simulink model "test_mdl_NI"  (R2018a)
settings: Solver=VariableStepAuto  StartTime=0.0  StopTime=10.0  RelTol=1e-3
(part 1 of 24)
settings Model: Creator=MSHI15  LastModifiedBy=MSHI15

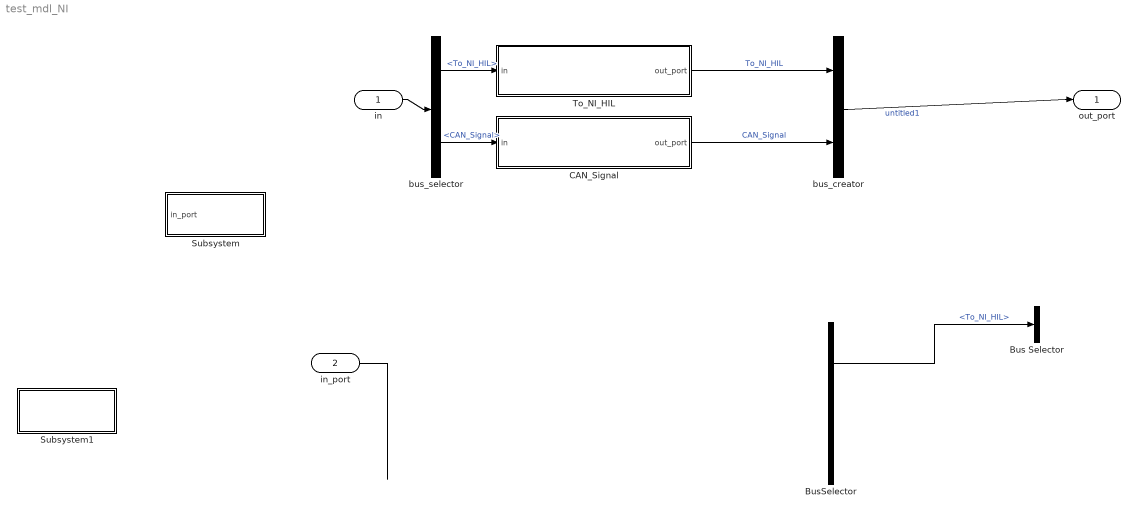
== system test_mdl_NI ==
  in : Inport
  in_port : Inport  Port=2
  Bus Selector : BusSelector  OutputSignals=signal1,signal2
  BusSelector : BusSelector  OutputSignals=To_NI_HIL,CAN_Signal
  CAN_Signal : Subsystem
  Subsystem : Subsystem
  Subsystem1 : Subsystem
  To_NI_HIL : Subsystem
  bus_creator : BusCreator  Inputs=2
  bus_selector : BusSelector  OutputSignals=To_NI_HIL,CAN_Signal
  out_port : Outport
  wires:
  BusSelector/1 -> Bus Selector/1  "<To_NI_HIL>"
  bus_creator/1 -> out_port/1  "untitled1"
  To_NI_HIL/1(out_port) -> bus_creator/1  "To_NI_HIL"
  CAN_Signal/1(out_port) -> bus_creator/2  "CAN_Signal"
  bus_selector/1 -> To_NI_HIL/1(in)  "<To_NI_HIL>"
  bus_selector/2 -> CAN_Signal/1(in)  "<CAN_Signal>"
  in/1 -> bus_selector/1
  in_port/1 -> ?

== system test_mdl_NI/CAN_Signal ==
  in : Inport
  ABS_ESC : Subsystem
  ADAS : Subsystem
  BCM : Subsystem
  DSMC : Subsystem
  ECM_DIESEL PCM PCM_HEV : Subsystem
  GWM : Subsystem
  PSCM : Subsystem
  RealPCM : Subsystem
  bus_creator : BusCreator  Inputs=8
  bus_selector : BusSelector  OutputSignals=ADAS,RealPCM,ABS_ESC,PSCM,ECM_DIESEL PCM PCM_HEV,BCM,GWM,DSMC
  out_port : Outport
  wires:
  bus_creator/1 -> out_port/1  "CAN_Signal"
  ADAS/1(out_port) -> bus_creator/1  "ADAS"
  RealPCM/1(out_port) -> bus_creator/2  "RealPCM"
  ABS_ESC/1(out_port) -> bus_creator/3  "ABS_ESC"
  PSCM/1(out_port) -> bus_creator/4  "PSCM"
  BCM/1(out_port) -> bus_creator/6  "BCM"
  GWM/1(out_port) -> bus_creator/7  "GWM"
  DSMC/1(out_port) -> bus_creator/8  "DSMC"
  ECM_DIESEL PCM PCM_HEV/1(out_port) -> bus_creator/5  "ECM_DIESEL PCM PCM_HEV"
  bus_selector/1 -> ADAS/1(in)  "<ADAS>"
  bus_selector/2 -> RealPCM/1(in)  "<RealPCM>"
  bus_selector/3 -> ABS_ESC/1(in)  "<ABS_ESC>"
  bus_selector/4 -> PSCM/1(in)  "<PSCM>"
  bus_selector/5 -> ECM_DIESEL PCM PCM_HEV/1(in)  "<ECM_DIESEL PCM PCM_HEV>"
  bus_selector/6 -> BCM/1(in)  "<BCM>"
  bus_selector/7 -> GWM/1(in)  "<GWM>"
  bus_selector/8 -> DSMC/1(in)  "<DSMC>"
  in/1 -> bus_selector/1

== system test_mdl_NI/Subsystem ==
  in_port : Inport
  ABS_ESC : Subsystem
  CMR_DSMC : Subsystem
  ECM_Diesel : Subsystem
  GWM : Subsystem
  IPMA_ADAS : Subsystem
  PCM : Subsystem
  PCM_HEV : Subsystem
  PSCM : Subsystem
  SOBDMC_HPCM_FD1 : Subsystem
  TCCM : Subsystem
  TCM_DSL : Subsystem
  TSTR : Subsystem
  VDM : Subsystem
  bus_selector : BusSelector  OutputSignals=ABS_ESC,CMR_DSMC,ECM_Diesel,GWM,IPMA_ADAS,PCM,PCM_HEV,PSCM,SOBDMC_HPCM_FD1,TCCM,TCM_DSL,TSTR,VDM
  wires:
  in_port/1 -> bus_selector/1  "Subsystem"
  bus_selector/1 -> ABS_ESC/1(in_port)  "<ABS_ESC>"
  bus_selector/2 -> CMR_DSMC/1(in_port)  "<CMR_DSMC>"
  bus_selector/3 -> ECM_Diesel/1(in_port)  "<ECM_Diesel>"
  bus_selector/4 -> GWM/1(in_port)  "<GWM>"
  bus_selector/5 -> IPMA_ADAS/1(in_port)  "<IPMA_ADAS>"
  bus_selector/6 -> PCM/1(in_port)  "<PCM>"
  bus_selector/7 -> PCM_HEV/1(in_port)  "<PCM_HEV>"
  bus_selector/8 -> PSCM/1(in_port)  "<PSCM>"
  bus_selector/9 -> SOBDMC_HPCM_FD1/1(in_port)  "<SOBDMC_HPCM_FD1>"
  bus_selector/10 -> TCCM/1(in_port)  "<TCCM>"
  bus_selector/11 -> TCM_DSL/1(in_port)  "<TCM_DSL>"
  bus_selector/12 -> TSTR/1(in_port)  "<TSTR>"
  bus_selector/13 -> VDM/1(in_port)  "<VDM>"

== system test_mdl_NI/Subsystem1 ==

== system test_mdl_NI/To_NI_HIL ==
  in : Inport
  DSMC : Subsystem
  MRR : Subsystem
  SRR_L : Subsystem
  SRR_R : Subsystem
  Soft_ABS : Subsystem
  Soft_APIM : Subsystem
  Soft_BCM : Subsystem
  Soft_CCM : Subsystem
  Soft_ECM : Subsystem
  Soft_IPC : Subsystem
  Soft_IPMA : Subsystem
  Soft_MRR : Subsystem
  Soft_PCM : Subsystem
  Soft_PSCM : Subsystem
  Soft_RCM : Subsystem
  Soft_SCCM : Subsystem
  Soft_TCM : Subsystem
  bus_creator : BusCreator  Inputs=17
  bus_selector : BusSelector  OutputSignals=Soft_ABS,Soft_PCM,Soft_ECM,Soft_TCM,Soft_PSCM,Soft_RCM,Soft_SCCM,Soft_MRR,Soft_BCM,Soft_IPC,Soft_APIM,Soft_IPMA,Soft_CCM,MRR,SRR_R,SRR_L,DSMC
  out_port : Outport
  wires:
  bus_creator/1 -> out_port/1  "To_NI_HIL"
  Soft_IPC/1(out) -> bus_creator/10  "Soft_IPC"
  Soft_APIM/1(out) -> bus_creator/11  "Soft_APIM"
  Soft_IPMA/1(out) -> bus_creator/12  "Soft_IPMA"
  Soft_CCM/1(out) -> bus_creator/13  "Soft_CCM"
  Soft_ABS/1(out_port) -> bus_creator/1  "Soft_ABS"
  Soft_PCM/1(out_port) -> bus_creator/2  "Soft_PCM"
  Soft_ECM/1(out_port) -> bus_creator/3  "Soft_ECM"
  Soft_TCM/1(out_port) -> bus_creator/4  "Soft_TCM"
  Soft_PSCM/1(out_port) -> bus_creator/5  "Soft_PSCM"
  Soft_RCM/1(out_port) -> bus_creator/6  "Soft_RCM"
  Soft_SCCM/1(out_port) -> bus_creator/7  "Soft_SCCM"
  Soft_MRR/1(out_port) -> bus_creator/8  "Soft_MRR"
  Soft_BCM/1(out_port) -> bus_creator/9  "Soft_BCM"
  MRR/1(out_port) -> bus_creator/14  "MRR"
  SRR_R/1(out_port) -> bus_creator/15  "SRR_R"
  SRR_L/1(out_port) -> bus_creator/16  "SRR_L"
  DSMC/1(out_port) -> bus_creator/17  "DSMC"
  bus_selector/1 -> Soft_ABS/1(in)  "<Soft_ABS>"
  bus_selector/2 -> Soft_PCM/1(in)  "<Soft_PCM>"
  bus_selector/3 -> Soft_ECM/1(in)  "<Soft_ECM>"
  bus_selector/4 -> Soft_TCM/1(in)  "<Soft_TCM>"
  bus_selector/5 -> Soft_PSCM/1(in)  "<Soft_PSCM>"
  bus_selector/6 -> Soft_RCM/1(in)  "<Soft_RCM>"
  bus_selector/7 -> Soft_SCCM/1(in)  "<Soft_SCCM>"
  bus_selector/8 -> Soft_MRR/1(in)  "<Soft_MRR>"
  bus_selector/9 -> Soft_BCM/1(in)  "<Soft_BCM>"
  bus_selector/10 -> Soft_IPC/1(in)  "<Soft_IPC>"
  bus_selector/11 -> Soft_APIM/1(in)  "<Soft_APIM>"
  bus_selector/12 -> Soft_IPMA/1(in)  "<Soft_IPMA>"
  bus_selector/13 -> Soft_CCM/1(in)  "<Soft_CCM>"
  bus_selector/14 -> MRR/1(in)  "<MRR>"
  bus_selector/15 -> SRR_R/1(in)  "<SRR_R>"
  bus_selector/16 -> SRR_L/1(in)  "<SRR_L>"
  bus_selector/17 -> DSMC/1(in)  "<DSMC>"
  in/1 -> bus_selector/1

== system test_mdl_NI/CAN_Signal/ABS_ESC ==
  in : Inport
  ABS_AutoSar_NetworkMgt_0x596 : Subsystem
  ABS_BrkBst_Data_0x4B0 : Subsystem
  ABS_Rapid_Data_Response_1_0x6B0 : Subsystem
  ABS_Rapid_Data_Response_2_0x6B1 : Subsystem
  ActiveFronSteering_Req_0x88 : Subsystem
  BrakeSnData_3_0x77 : Subsystem
  BrakeSnData_4_0x7D : Subsystem
  BrakeSnData_5_0x76 : Subsystem
  BrakeSnData_6_0x414 : Subsystem
  BrakeSysFeatures_0x415 : Subsystem
  BrakeSysFeatures_2_0x416 : Subsystem
  BrakeSysFeatures_3_0x41E : Subsystem
  DesiredTorqBrk_0x213 : Subsystem
  DesiredTorqBrk_2_0x214 : Subsystem
  Global_PATS_SubTarget_0x49 : Subsystem
  SelectDriveModeData2_0x44E : Subsystem
  SelectDriveModeData_0x420 : Subsystem
  SteeringPinion_Data2_0x7F : Subsystem
  TesterPhysicalResABS_0x768 : Subsystem
  TrailerBrakeData_0x412 : Subsystem
  WheelData_0x216 : Subsystem
  WheelSpeed_0x217 : Subsystem
  bus_creator : BusCreator  Inputs=22
  bus_selector : BusSelector  OutputSignals=Global_PATS_SubTarget_0x49,BrakeSnData_5_0x76,BrakeSnData_3_0x77,BrakeSnData_4_0x7D,SteeringPinion_Data2_0x7F,ActiveFronSteering_Req_0x88,DesiredTorqBrk_0x213,DesiredTorqBrk_2_0x214,WheelData_0x216,WheelSpeed_0x217,TrailerBrakeData_0x412,BrakeSnData_6_0x414,BrakeSysFeatures_0x415,BrakeSysFeatures_2_0x416,BrakeSysFeatures_3_0x41E,SelectDriveModeData_0x420,SelectDriveModeData2_0x44E,ABS_BrkBst_Data_0x4B0,ABS_AutoSar_NetworkMgt_0x596,ABS_Rapid_Data_Response_1_0x6B0,ABS_Rapid_Data_Response_2_0x6B1,TesterPhysicalResABS_0x768
  out_port : Outport
  wires:
  bus_creator/1 -> out_port/1  "ABS_ESC"
  Global_PATS_SubTarget_0x49/1(out_port) -> bus_creator/1  "Global_PATS_SubTarget_0x49"
  BrakeSnData_5_0x76/1(out_port) -> bus_creator/2  "BrakeSnData_5_0x76"
  BrakeSnData_3_0x77/1(out_port) -> bus_creator/3  "BrakeSnData_3_0x77"
  BrakeSnData_4_0x7D/1(out_port) -> bus_creator/4  "BrakeSnData_4_0x7D"
  SteeringPinion_Data2_0x7F/1(out_port) -> bus_creator/5  "SteeringPinion_Data2_0x7F"
  ActiveFronSteering_Req_0x88/1(out_port) -> bus_creator/6  "ActiveFronSteering_Req_0x88"
  DesiredTorqBrk_0x213/1(out_port) -> bus_creator/7  "DesiredTorqBrk_0x213"
  DesiredTorqBrk_2_0x214/1(out_port) -> bus_creator/8  "DesiredTorqBrk_2_0x214"
  WheelData_0x216/1(out_port) -> bus_creator/9  "WheelData_0x216"
  WheelSpeed_0x217/1(out_port) -> bus_creator/10  "WheelSpeed_0x217"
  TrailerBrakeData_0x412/1(out_port) -> bus_creator/11  "TrailerBrakeData_0x412"
  BrakeSnData_6_0x414/1(out_port) -> bus_creator/12  "BrakeSnData_6_0x414"
  BrakeSysFeatures_0x415/1(out_port) -> bus_creator/13  "BrakeSysFeatures_0x415"
  BrakeSysFeatures_2_0x416/1(out_port) -> bus_creator/14  "BrakeSysFeatures_2_0x416"
  BrakeSysFeatures_3_0x41E/1(out_port) -> bus_creator/15  "BrakeSysFeatures_3_0x41E"
  SelectDriveModeData_0x420/1(out_port) -> bus_creator/16  "SelectDriveModeData_0x420"
  SelectDriveModeData2_0x44E/1(out_port) -> bus_creator/17  "SelectDriveModeData2_0x44E"
  ABS_BrkBst_Data_0x4B0/1(out_port) -> bus_creator/18  "ABS_BrkBst_Data_0x4B0"
  ABS_AutoSar_NetworkMgt_0x596/1(out_port) -> bus_creator/19  "ABS_AutoSar_NetworkMgt_0x596"
  ABS_Rapid_Data_Response_1_0x6B0/1(out_port) -> bus_creator/20  "ABS_Rapid_Data_Response_1_0x6B0"
  ABS_Rapid_Data_Response_2_0x6B1/1(out_port) -> bus_creator/21  "ABS_Rapid_Data_Response_2_0x6B1"
  TesterPhysicalResABS_0x768/1(out_port) -> bus_creator/22  "TesterPhysicalResABS_0x768"
  bus_selector/1 -> Global_PATS_SubTarget_0x49/1(in)  "<Global_PATS_SubTarget_0x49>"
  bus_selector/2 -> BrakeSnData_5_0x76/1(in)  "<BrakeSnData_5_0x76>"
  bus_selector/3 -> BrakeSnData_3_0x77/1(in)  "<BrakeSnData_3_0x77>"
  bus_selector/4 -> BrakeSnData_4_0x7D/1(in)  "<BrakeSnData_4_0x7D>"
  bus_selector/5 -> SteeringPinion_Data2_0x7F/1(in)  "<SteeringPinion_Data2_0x7F>"
  bus_selector/6 -> ActiveFronSteering_Req_0x88/1(in)  "<ActiveFronSteering_Req_0x88>"
  bus_selector/7 -> DesiredTorqBrk_0x213/1(in)  "<DesiredTorqBrk_0x213>"
  bus_selector/8 -> DesiredTorqBrk_2_0x214/1(in)  "<DesiredTorqBrk_2_0x214>"
  bus_selector/9 -> WheelData_0x216/1(in)  "<WheelData_0x216>"
  bus_selector/10 -> WheelSpeed_0x217/1(in)  "<WheelSpeed_0x217>"
  bus_selector/11 -> TrailerBrakeData_0x412/1(in)  "<TrailerBrakeData_0x412>"
  bus_selector/12 -> BrakeSnData_6_0x414/1(in)  "<BrakeSnData_6_0x414>"
  bus_selector/13 -> BrakeSysFeatures_0x415/1(in)  "<BrakeSysFeatures_0x415>"
  bus_selector/14 -> BrakeSysFeatures_2_0x416/1(in)  "<BrakeSysFeatures_2_0x416>"
  bus_selector/15 -> BrakeSysFeatures_3_0x41E/1(in)  "<BrakeSysFeatures_3_0x41E>"
  bus_selector/16 -> SelectDriveModeData_0x420/1(in)  "<SelectDriveModeData_0x420>"
  bus_selector/17 -> SelectDriveModeData2_0x44E/1(in)  "<SelectDriveModeData2_0x44E>"
  bus_selector/18 -> ABS_BrkBst_Data_0x4B0/1(in)  "<ABS_BrkBst_Data_0x4B0>"
  bus_selector/19 -> ABS_AutoSar_NetworkMgt_0x596/1(in)  "<ABS_AutoSar_NetworkMgt_0x596>"
  bus_selector/20 -> ABS_Rapid_Data_Response_1_0x6B0/1(in)  "<ABS_Rapid_Data_Response_1_0x6B0>"
  bus_selector/21 -> ABS_Rapid_Data_Response_2_0x6B1/1(in)  "<ABS_Rapid_Data_Response_2_0x6B1>"
  bus_selector/22 -> TesterPhysicalResABS_0x768/1(in)  "<TesterPhysicalResABS_0x768>"
  in/1 -> bus_selector/1

== system test_mdl_NI/CAN_Signal/ADAS ==
  in : Inport
  ACCDATA : Subsystem
  ACCDATA_2 : Subsystem
  bus_creator : BusCreator  Inputs=2
  bus_selector : BusSelector  OutputSignals=ACCDATA,ACCDATA_2
  out_port : Outport
  wires:
  bus_creator/1 -> out_port/1  "ADAS"
  ACCDATA/1(out_port) -> bus_creator/1  "ACCDATA"
  ACCDATA_2/1(out_port) -> bus_creator/2  "ACCDATA_2"
  bus_selector/1 -> ACCDATA/1(in)  "<ACCDATA>"
  bus_selector/2 -> ACCDATA_2/1(in)  "<ACCDATA_2>"
  in/1 -> bus_selector/1

== system test_mdl_NI/CAN_Signal/BCM ==
  in : Inport
  BCM_Lamp_Stat_0x3C3 : Subsystem
  Battery_Mgmt_24V_0x42E : Subsystem
  Battery_Mgmt_2_0x42C : Subsystem
  Battery_Mgmt_3_0x43C : Subsystem
  Battery_Mgmt_4_0x42B : Subsystem
  BodyInfo_3_0x3B3 : Subsystem
  Body_Info_10_0x3BA : Subsystem
  Body_Info_12_0x26E : Subsystem
  Body_Info_4_0x242 : Subsystem
  Body_Info_6_0x38D : Subsystem
  Body_Info_7_0x3B1 : Subsystem
  Body_Info_8_0x3B9 : Subsystem
  Body_Info_9_0x3A3 : Subsystem
  CMPS_FDM_Info_Status_0x3C7 : Subsystem
  CellPhonePassport_Stat_1_0x447 : Subsystem
  GGCC_Config_Mgmt_ID_1_0x40A : Subsystem
  GlobalClock_Data_0x84 : Subsystem
  Global_PATS_Control_Info2_0x42 : Subsystem
  Global_PATS_Control_Info_0x41 : Subsystem
  Locking_Systems_2_0x331 : Subsystem
  PaakRqData1_0x468 : Subsystem
  PaakRqData2_0x469 : Subsystem
  Personality_BCM2_Data_0x3EB : Subsystem
  Personality_BCM_Data_0x3E3 : Subsystem
  Power_Stat_0x456 : Subsystem
  RKE_Packet_0x3B6 : Subsystem
  TPM_Frame_0x3B7 : Subsystem
  Tire_Pressure_Data_0x3B5 : Subsystem
  Tire_Pressure_Data_DRW_0x3B8 : Subsystem
  Tire_Pressure_Stat_0x3B4 : Subsystem
  bus_creator : BusCreator  Inputs=30
  bus_selector : BusSelector  OutputSignals=Global_PATS_Control_Info_0x41,Global_PATS_Control_Info2_0x42,GlobalClock_Data_0x84,Body_Info_4_0x242,Body_Info_12_0x26E,Locking_Systems_2_0x331,Body_Info_6_0x38D,Body_Info_9_0x3A3,Body_Info_7_0x3B1,BodyInfo_3_0x3B3,Tire_Pressure_Stat_0x3B4,Tire_Pressure_Data_0x3B5,RKE_Packet_0x3B6,TPM_Frame_0x3B7,Tire_Pressure_Data_DRW_0x3B8,Body_Info_8_0x3B9,Body_Info_10_0x3BA,BCM_Lamp_Stat_0x3C3,CMPS_FDM_Info_Status_0x3C7,Personality_BCM_Data_0x3E3,Personality_BCM2_Data_0x3EB,GGCC_Config_Mgmt_ID_1_0x40A,Battery_Mgmt_4_0x42B,Battery_Mgmt_2_0x42C,Battery_Mgmt_24V_0x42E,Battery_Mgmt_3_0x43C,CellPhonePassport_Stat_1_0x447,Power_Stat_0x456,PaakRqData1_0x468,PaakRqData2_0x469
  out_port : Outport
  wires:
  bus_creator/1 -> out_port/1  "BCM"
  Global_PATS_Control_Info_0x41/1(out_port) -> bus_creator/1  "Global_PATS_Control_Info_0x41"
  Global_PATS_Control_Info2_0x42/1(out_port) -> bus_creator/2  "Global_PATS_Control_Info2_0x42"
  GlobalClock_Data_0x84/1(out_port) -> bus_creator/3  "GlobalClock_Data_0x84"
  Body_Info_4_0x242/1(out_port) -> bus_creator/4  "Body_Info_4_0x242"
  Body_Info_12_0x26E/1(out_port) -> bus_creator/5  "Body_Info_12_0x26E"
  Locking_Systems_2_0x331/1(out_port) -> bus_creator/6  "Locking_Systems_2_0x331"
  Body_Info_6_0x38D/1(out_port) -> bus_creator/7  "Body_Info_6_0x38D"
  Body_Info_9_0x3A3/1(out_port) -> bus_creator/8  "Body_Info_9_0x3A3"
  Body_Info_7_0x3B1/1(out_port) -> bus_creator/9  "Body_Info_7_0x3B1"
  BodyInfo_3_0x3B3/1(out_port) -> bus_creator/10  "BodyInfo_3_0x3B3"
  Tire_Pressure_Stat_0x3B4/1(out_port) -> bus_creator/11  "Tire_Pressure_Stat_0x3B4"
  Tire_Pressure_Data_0x3B5/1(out_port) -> bus_creator/12  "Tire_Pressure_Data_0x3B5"
  RKE_Packet_0x3B6/1(out_port) -> bus_creator/13  "RKE_Packet_0x3B6"
  TPM_Frame_0x3B7/1(out_port) -> bus_creator/14  "TPM_Frame_0x3B7"
  Tire_Pressure_Data_DRW_0x3B8/1(out_port) -> bus_creator/15  "Tire_Pressure_Data_DRW_0x3B8"
  Body_Info_8_0x3B9/1(out_port) -> bus_creator/16  "Body_Info_8_0x3B9"
  Body_Info_10_0x3BA/1(out_port) -> bus_creator/17  "Body_Info_10_0x3BA"
  BCM_Lamp_Stat_0x3C3/1(out_port) -> bus_creator/18  "BCM_Lamp_Stat_0x3C3"
  CMPS_FDM_Info_Status_0x3C7/1(out_port) -> bus_creator/19  "CMPS_FDM_Info_Status_0x3C7"
  Personality_BCM_Data_0x3E3/1(out_port) -> bus_creator/20  "Personality_BCM_Data_0x3E3"
  Personality_BCM2_Data_0x3EB/1(out_port) -> bus_creator/21  "Personality_BCM2_Data_0x3EB"
  GGCC_Config_Mgmt_ID_1_0x40A/1(out_port) -> bus_creator/22  "GGCC_Config_Mgmt_ID_1_0x40A"
  Battery_Mgmt_4_0x42B/1(out_port) -> bus_creator/23  "Battery_Mgmt_4_0x42B"
  Battery_Mgmt_2_0x42C/1(out_port) -> bus_creator/24  "Battery_Mgmt_2_0x42C"
  Battery_Mgmt_24V_0x42E/1(out_port) -> bus_creator/25  "Battery_Mgmt_24V_0x42E"
  Battery_Mgmt_3_0x43C/1(out_port) -> bus_creator/26  "Battery_Mgmt_3_0x43C"
  CellPhonePassport_Stat_1_0x447/1(out_port) -> bus_creator/27  "CellPhonePassport_Stat_1_0x447"
  Power_Stat_0x456/1(out_port) -> bus_creator/28  "Power_Stat_0x456"
  PaakRqData1_0x468/1(out_port) -> bus_creator/29  "PaakRqData1_0x468"
  PaakRqData2_0x469/1(out_port) -> bus_creator/30  "PaakRqData2_0x469"
  bus_selector/1 -> Global_PATS_Control_Info_0x41/1(in)  "<Global_PATS_Control_Info_0x41>"
  bus_selector/2 -> Global_PATS_Control_Info2_0x42/1(in)  "<Global_PATS_Control_Info2_0x42>"
  bus_selector/3 -> GlobalClock_Data_0x84/1(in)  "<GlobalClock_Data_0x84>"
  bus_selector/4 -> Body_Info_4_0x242/1(in)  "<Body_Info_4_0x242>"
  bus_selector/5 -> Body_Info_12_0x26E/1(in)  "<Body_Info_12_0x26E>"
  bus_selector/6 -> Locking_Systems_2_0x331/1(in)  "<Locking_Systems_2_0x331>"
  bus_selector/7 -> Body_Info_6_0x38D/1(in)  "<Body_Info_6_0x38D>"
  bus_selector/8 -> Body_Info_9_0x3A3/1(in)  "<Body_Info_9_0x3A3>"
  bus_selector/9 -> Body_Info_7_0x3B1/1(in)  "<Body_Info_7_0x3B1>"
  bus_selector/10 -> BodyInfo_3_0x3B3/1(in)  "<BodyInfo_3_0x3B3>"
  bus_selector/11 -> Tire_Pressure_Stat_0x3B4/1(in)  "<Tire_Pressure_Stat_0x3B4>"
  bus_selector/12 -> Tire_Pressure_Data_0x3B5/1(in)  "<Tire_Pressure_Data_0x3B5>"
  bus_selector/13 -> RKE_Packet_0x3B6/1(in)  "<RKE_Packet_0x3B6>"
  bus_selector/14 -> TPM_Frame_0x3B7/1(in)  "<TPM_Frame_0x3B7>"
  bus_selector/15 -> Tire_Pressure_Data_DRW_0x3B8/1(in)  "<Tire_Pressure_Data_DRW_0x3B8>"
  bus_selector/16 -> Body_Info_8_0x3B9/1(in)  "<Body_Info_8_0x3B9>"
  bus_selector/17 -> Body_Info_10_0x3BA/1(in)  "<Body_Info_10_0x3BA>"
  bus_selector/18 -> BCM_Lamp_Stat_0x3C3/1(in)  "<BCM_Lamp_Stat_0x3C3>"
  bus_selector/19 -> CMPS_FDM_Info_Status_0x3C7/1(in)  "<CMPS_FDM_Info_Status_0x3C7>"
  bus_selector/20 -> Personality_BCM_Data_0x3E3/1(in)  "<Personality_BCM_Data_0x3E3>"
  bus_selector/21 -> Personality_BCM2_Data_0x3EB/1(in)  "<Personality_BCM2_Data_0x3EB>"
  bus_selector/22 -> GGCC_Config_Mgmt_ID_1_0x40A/1(in)  "<GGCC_Config_Mgmt_ID_1_0x40A>"
  bus_selector/23 -> Battery_Mgmt_4_0x42B/1(in)  "<Battery_Mgmt_4_0x42B>"
  bus_selector/24 -> Battery_Mgmt_2_0x42C/1(in)  "<Battery_Mgmt_2_0x42C>"
  bus_selector/25 -> Battery_Mgmt_24V_0x42E/1(in)  "<Battery_Mgmt_24V_0x42E>"
  bus_selector/26 -> Battery_Mgmt_3_0x43C/1(in)  "<Battery_Mgmt_3_0x43C>"
  bus_selector/27 -> CellPhonePassport_Stat_1_0x447/1(in)  "<CellPhonePassport_Stat_1_0x447>"
  bus_selector/28 -> Power_Stat_0x456/1(in)  "<Power_Stat_0x456>"
  bus_selector/29 -> PaakRqData1_0x468/1(in)  "<PaakRqData1_0x468>"
  bus_selector/30 -> PaakRqData2_0x469/1(in)  "<PaakRqData2_0x469>"
  in/1 -> bus_selector/1

== system test_mdl_NI/CAN_Signal/DSMC ==
  in : Inport
  CMR_DSMC_AutoSar_NetwrkMgt : Subsystem
  DrvStatMonData : Subsystem
  TesterPhysicalResCMR_DSMC : Subsystem
  bus_creator : BusCreator  Inputs=3
  bus_selector : BusSelector  OutputSignals=CMR_DSMC_AutoSar_NetwrkMgt,DrvStatMonData,TesterPhysicalResCMR_DSMC
  out_port : Outport
  wires:
  bus_creator/1 -> out_port/1  "DSMC"
  CMR_DSMC_AutoSar_NetwrkMgt/1(out_port) -> bus_creator/1  "CMR_DSMC_AutoSar_NetwrkMgt"
  DrvStatMonData/1(out_port) -> bus_creator/2  "DrvStatMonData"
  TesterPhysicalResCMR_DSMC/1(out_port) -> bus_creator/3  "TesterPhysicalResCMR_DSMC"
  bus_selector/1 -> CMR_DSMC_AutoSar_NetwrkMgt/1(in)  "<CMR_DSMC_AutoSar_NetwrkMgt>"
  bus_selector/2 -> DrvStatMonData/1(in)  "<DrvStatMonData>"
  bus_selector/3 -> TesterPhysicalResCMR_DSMC/1(in)  "<TesterPhysicalResCMR_DSMC>"
  in/1 -> bus_selector/1

== system test_mdl_NI/CAN_Signal/ECM_DIESEL PCM PCM_HEV ==
  in : Inport
  EngBrakeData_0x165 : Subsystem
  EngVehicleSpThrottle2_0x202 : Subsystem
  EngVehicleSpThrottle_0x204 : Subsystem
  EngineClimateData_0x178 : Subsystem
  EngineData_6_0x156 : Subsystem
  EngineData_7_0x179 : Subsystem
  Engine_Clutch_Data_0x42F : Subsystem
  Gear_Shift_by_Wire_3 : Subsystem
  Global_PATS_TargetInfo_0x47 : Subsystem
  HEV_Powertrain_Data2 : Subsystem
  PCM_AutoSar_NetworkMgmt_0x595 : Subsystem
  PCM_Rapid_Data_Response_1_0x6A0 : Subsystem
  PowertrainData_10 : Subsystem
  PowertrainData_1_0x421 : Subsystem
  PowertrainData_2_0x42D : Subsystem
  PowertrainData_3_0x43E : Subsystem
  PowertrainData_6_0x205 : Subsystem
  PowertrainData_7_0x41F : Subsystem
  PowertrainData_9_0x44C : Subsystem
  Powertrain_Data_4_0x424 : Subsystem
  Powertrain_Data_5_0x43F : Subsystem
  Stop_Start_0x166 : Subsystem
  TesterPhysicalResPCM_0x7E8 : Subsystem
  TorqueDataEngFlags_0x200 : Subsystem
  TransGearData : Subsystem
  VehicleOperatingModes_0x167 : Subsystem
  bus_creator : BusCreator  Inputs=26
  bus_selector : BusSelector  OutputSignals=Global_PATS_TargetInfo_0x47,EngineData_6_0x156,EngBrakeData_0x165,Stop_Start_0x166,VehicleOperatingModes_0x167,EngineClimateData_0x178,EngineData_7_0x179,TorqueDataEngFlags_0x200,EngVehicleSpThrottle2_0x202,EngVehicleSpThrottle_0x204,PowertrainData_6_0x205,PowertrainData_7_0x41F,PowertrainData_1_0x421,Powertrain_Data_4_0x424,PowertrainData_2_0x42D,Engine_Clutch_Data_0x42F,PowertrainData_3_0x43E,Powertrain_Data_5_0x43F,PowertrainData_9_0x44C,PCM_AutoSar_NetworkMgmt_0x595,PCM_Rapid_Data_Response_1_0x6A0,TesterPhysicalResPCM_0x7E8,Gear_Shift_by_Wire_3,PowertrainData_10,TransGearData,HEV_Powertrain_Data2
  out_port : Outport
  wires:
  bus_creator/1 -> out_port/1  "ECM_DIESEL PCM PCM_HEV"
  Global_PATS_TargetInfo_0x47/1(out_port) -> bus_creator/1  "Global_PATS_TargetInfo_0x47"
  EngineData_6_0x156/1(out_port) -> bus_creator/2  "EngineData_6_0x156"
  EngBrakeData_0x165/1(out_port) -> bus_creator/3  "EngBrakeData_0x165"
  Stop_Start_0x166/1(out_port) -> bus_creator/4  "Stop_Start_0x166"
  VehicleOperatingModes_0x167/1(out_port) -> bus_creator/5  "VehicleOperatingModes_0x167"
  EngineClimateData_0x178/1(out_port) -> bus_creator/6  "EngineClimateData_0x178"
  EngineData_7_0x179/1(out_port) -> bus_creator/7  "EngineData_7_0x179"
  TorqueDataEngFlags_0x200/1(out_port) -> bus_creator/8  "TorqueDataEngFlags_0x200"
  EngVehicleSpThrottle2_0x202/1(out_port) -> bus_creator/9  "EngVehicleSpThrottle2_0x202"
  EngVehicleSpThrottle_0x204/1(out_port) -> bus_creator/10  "EngVehicleSpThrottle_0x204"
  PowertrainData_6_0x205/1(out_port) -> bus_creator/11  "PowertrainData_6_0x205"
  PowertrainData_7_0x41F/1(out_port) -> bus_creator/12  "PowertrainData_7_0x41F"
  PowertrainData_1_0x421/1(out_port) -> bus_creator/13  "PowertrainData_1_0x421"
  Powertrain_Data_4_0x424/1(out_port) -> bus_creator/14  "Powertrain_Data_4_0x424"
  PowertrainData_2_0x42D/1(out_port) -> bus_creator/15  "PowertrainData_2_0x42D"
  Engine_Clutch_Data_0x42F/1(out_port) -> bus_creator/16  "Engine_Clutch_Data_0x42F"
  PowertrainData_3_0x43E/1(out_port) -> bus_creator/17  "PowertrainData_3_0x43E"
  Powertrain_Data_5_0x43F/1(out_port) -> bus_creator/18  "Powertrain_Data_5_0x43F"
  PowertrainData_9_0x44C/1(out_port) -> bus_creator/19  "PowertrainData_9_0x44C"
  PCM_AutoSar_NetworkMgmt_0x595/1(out_port) -> bus_creator/20  "PCM_AutoSar_NetworkMgmt_0x595"
  PCM_Rapid_Data_Response_1_0x6A0/1(out_port) -> bus_creator/21  "PCM_Rapid_Data_Response_1_0x6A0"
  TesterPhysicalResPCM_0x7E8/1(out_port) -> bus_creator/22  "TesterPhysicalResPCM_0x7E8"
  Gear_Shift_by_Wire_3/1(out_port) -> bus_creator/23  "Gear_Shift_by_Wire_3"
  PowertrainData_10/1(out_port) -> bus_creator/24  "PowertrainData_10"
  TransGearData/1(out_port) -> bus_creator/25  "TransGearData"
  HEV_Powertrain_Data2/1(out_port) -> bus_creator/26  "HEV_Powertrain_Data2"
  bus_selector/1 -> Global_PATS_TargetInfo_0x47/1(in)  "<Global_PATS_TargetInfo_0x47>"
  bus_selector/2 -> EngineData_6_0x156/1(in)  "<EngineData_6_0x156>"
  bus_selector/3 -> EngBrakeData_0x165/1(in)  "<EngBrakeData_0x165>"
  bus_selector/4 -> Stop_Start_0x166/1(in)  "<Stop_Start_0x166>"
  bus_selector/5 -> VehicleOperatingModes_0x167/1(in)  "<VehicleOperatingModes_0x167>"
  bus_selector/6 -> EngineClimateData_0x178/1(in)  "<EngineClimateData_0x178>"
  bus_selector/7 -> EngineData_7_0x179/1(in)  "<EngineData_7_0x179>"
  bus_selector/8 -> TorqueDataEngFlags_0x200/1(in)  "<TorqueDataEngFlags_0x200>"
  bus_selector/9 -> EngVehicleSpThrottle2_0x202/1(in)  "<EngVehicleSpThrottle2_0x202>"
  bus_selector/10 -> EngVehicleSpThrottle_0x204/1(in)  "<EngVehicleSpThrottle_0x204>"
  bus_selector/11 -> PowertrainData_6_0x205/1(in)  "<PowertrainData_6_0x205>"
  bus_selector/12 -> PowertrainData_7_0x41F/1(in)  "<PowertrainData_7_0x41F>"
  bus_selector/13 -> PowertrainData_1_0x421/1(in)  "<PowertrainData_1_0x421>"
  bus_selector/14 -> Powertrain_Data_4_0x424/1(in)  "<Powertrain_Data_4_0x424>"
  bus_selector/15 -> PowertrainData_2_0x42D/1(in)  "<PowertrainData_2_0x42D>"
  bus_selector/16 -> Engine_Clutch_Data_0x42F/1(in)  "<Engine_Clutch_Data_0x42F>"
  bus_selector/17 -> PowertrainData_3_0x43E/1(in)  "<PowertrainData_3_0x43E>"
  bus_selector/18 -> Powertrain_Data_5_0x43F/1(in)  "<Powertrain_Data_5_0x43F>"
  bus_selector/19 -> PowertrainData_9_0x44C/1(in)  "<PowertrainData_9_0x44C>"
  bus_selector/20 -> PCM_AutoSar_NetworkMgmt_0x595/1(in)  "<PCM_AutoSar_NetworkMgmt_0x595>"
  bus_selector/21 -> PCM_Rapid_Data_Response_1_0x6A0/1(in)  "<PCM_Rapid_Data_Response_1_0x6A0>"
  bus_selector/22 -> TesterPhysicalResPCM_0x7E8/1(in)  "<TesterPhysicalResPCM_0x7E8>"
  bus_selector/23 -> Gear_Shift_by_Wire_3/1(in)  "<Gear_Shift_by_Wire_3>"
  bus_selector/24 -> PowertrainData_10/1(in)  "<PowertrainData_10>"
  bus_selector/25 -> TransGearData/1(in)  "<TransGearData>"
  bus_selector/26 -> HEV_Powertrain_Data2/1(in)  "<HEV_Powertrain_Data2>"
  in/1 -> bus_selector/1

== system test_mdl_NI/CAN_Signal/GWM ==
  in : Inport
  GSM : Subsystem
  Other_GWMTx : Subsystem
  RCM : Subsystem
  SCCM : Subsystem
  Tester_AutoSar : Subsystem
  bus_creator : BusCreator  Inputs=5
  bus_selector : BusSelector  OutputSignals=Other_GWMTx,RCM,SCCM,GSM,Tester_AutoSar
  out_port : Outport
  wires:
  bus_creator/1 -> out_port/1  "GWM"
  Other_GWMTx/1(out_port) -> bus_creator/1  "Other_GWMTx"
  RCM/1(out_port) -> bus_creator/2  "RCM"
  SCCM/1(out_port) -> bus_creator/3  "SCCM"
  GSM/1(out_port) -> bus_creator/4  "GSM"
  Tester_AutoSar/1(out_port) -> bus_creator/5  "Tester_AutoSar"
  bus_selector/1 -> Other_GWMTx/1(in)  "<Other_GWMTx>"
  bus_selector/2 -> RCM/1(in)  "<RCM>"
  bus_selector/3 -> SCCM/1(in)  "<SCCM>"
  bus_selector/4 -> GSM/1(in)  "<GSM>"
  bus_selector/5 -> Tester_AutoSar/1(in)  "<Tester_AutoSar>"
  in/1 -> bus_selector/1

== system test_mdl_NI/CAN_Signal/PSCM ==
  in : Inport
  EPAS_INFO_0x82 : Subsystem
  Lane_Assist_Data3_FD1_0x3CC : Subsystem
  PSCM_AutoSar_NetwrkMgmt_0x5B5 : Subsystem
  SteeringPinion_Data_0x7E : Subsystem
  TesterPhysicalResPSCM_0x738 : Subsystem
  TrailerAid_Data2_0x417 : Subsystem
  bus_creator : BusCreator  Inputs=6
  bus_selector : BusSelector  OutputSignals=SteeringPinion_Data_0x7E,EPAS_INFO_0x82,Lane_Assist_Data3_FD1_0x3CC,TrailerAid_Data2_0x417,PSCM_AutoSar_NetwrkMgmt_0x5B5,TesterPhysicalResPSCM_0x738
  out_port : Outport
  wires:
  bus_creator/1 -> out_port/1  "PSCM"
  SteeringPinion_Data_0x7E/1(out_port) -> bus_creator/1  "SteeringPinion_Data_0x7E"
  EPAS_INFO_0x82/1(out_port) -> bus_creator/2  "EPAS_INFO_0x82"
  Lane_Assist_Data3_FD1_0x3CC/1(out_port) -> bus_creator/3  "Lane_Assist_Data3_FD1_0x3CC"
  TrailerAid_Data2_0x417/1(out_port) -> bus_creator/4  "TrailerAid_Data2_0x417"
  PSCM_AutoSar_NetwrkMgmt_0x5B5/1(out_port) -> bus_creator/5  "PSCM_AutoSar_NetwrkMgmt_0x5B5"
  TesterPhysicalResPSCM_0x738/1(out_port) -> bus_creator/6  "TesterPhysicalResPSCM_0x738"
  bus_selector/1 -> SteeringPinion_Data_0x7E/1(in)  "<SteeringPinion_Data_0x7E>"
  bus_selector/2 -> EPAS_INFO_0x82/1(in)  "<EPAS_INFO_0x82>"
  bus_selector/3 -> Lane_Assist_Data3_FD1_0x3CC/1(in)  "<Lane_Assist_Data3_FD1_0x3CC>"
  bus_selector/4 -> TrailerAid_Data2_0x417/1(in)  "<TrailerAid_Data2_0x417>"
  bus_selector/5 -> PSCM_AutoSar_NetwrkMgmt_0x5B5/1(in)  "<PSCM_AutoSar_NetwrkMgmt_0x5B5>"
  bus_selector/6 -> TesterPhysicalResPSCM_0x738/1(in)  "<TesterPhysicalResPSCM_0x738>"
  in/1 -> bus_selector/1

== system test_mdl_NI/CAN_Signal/RealPCM ==
  in : Inport
  EngBrakeData : Subsystem
  EngVehicleSpThrottle2 : Subsystem
  bus_creator : BusCreator  Inputs=3
  bus_selector : BusSelector  OutputSignals=EngBrakeData,EngVehicleSpThrottle2,user_channel
  user_channel : Subsystem
  out_port : Outport
  wires:
  bus_creator/1 -> out_port/1  "RealPCM"
  EngBrakeData/1(out_port) -> bus_creator/1  "EngBrakeData"
  EngVehicleSpThrottle2/1(out_port) -> bus_creator/2  "EngVehicleSpThrottle2"
  user_channel/1(out_port) -> bus_creator/3  "user_channel"
  bus_selector/1 -> EngBrakeData/1(in)  "<EngBrakeData>"
  bus_selector/2 -> EngVehicleSpThrottle2/1(in)  "<EngVehicleSpThrottle2>"
  bus_selector/3 -> user_channel/1(in)  "<user_channel>"
  in/1 -> bus_selector/1

== system test_mdl_NI/Subsystem/ABS_ESC ==
  in_port : Inport
  ABS_AutoSar_NetworkMgt_Ox596 : Subsystem
  ABS_BrkBst_Data_Ox4B0 : Subsystem
  ABS_Rapid_Data_Response_1_Ox6B0 : Subsystem
  ABS_Rapid_Data_Response_2_Ox6B1 : Subsystem
  ActiveFronSteering_Req_Ox88 : Subsystem
  BrakeSnData_3_Ox77 : Subsystem
  BrakeSnData_4_Ox7D : Subsystem
  BrakeSnData_5_Ox76 : Subsystem
  BrakeSnData_6_Ox414 : Subsystem
  BrakeSysFeatures_2_Ox416 : Subsystem
  BrakeSysFeatures_3_Ox41E : Subsystem
  BrakeSysFeatures_Ox415 : Subsystem
  DesiredTorqBrk_2_Ox214 : Subsystem
  DesiredTorqBrk_Ox213 : Subsystem
  Global_PATS_SubTarget_Ox49 : Subsystem
  OTAPhysABStoGWM_ECG_Ox1B936028 : Subsystem
  PARSEDPhysABStoGWM_ECG_Ox1BA36028 : Subsystem
  PARSEDPushABStoGWM_ECG_Ox1BB36028 : Subsystem
  SelectDriveModeData2_Ox44E : Subsystem
  SelectDriveModeData_Ox420 : Subsystem
  TesterPhysicalResABS_Ox768 : Subsystem
  TrailerBrakeData_Ox412 : Subsystem
  WheelData_Ox216 : Subsystem
  WheelSpeed_Ox217 : Subsystem
  bus_selector : BusSelector  OutputSignals=ABS_AutoSar_NetworkMgt_Ox596,ABS_BrkBst_Data_Ox4B0,ABS_Rapid_Data_Response_1_Ox6B0,ABS_Rapid_Data_Response_2_Ox6B1,ActiveFronSteering_Req_Ox88,BrakeSnData_3_Ox77,BrakeSnData_4_Ox7D,BrakeSnData_5_Ox76,BrakeSnData_6_Ox414,BrakeSysFeatures_Ox415,BrakeSysFeatures_2_Ox416,BrakeSysFeatures_3_Ox41E,DesiredTorqBrk_Ox213,DesiredTorqBrk_2_Ox214,Global_PATS_SubTarget_Ox49,OTAPhysABStoGWM_ECG_Ox1B936028,PARSEDPhysABStoGWM_ECG_Ox1BA36028,PARSEDPushABStoGWM_ECG_Ox1BB36028,SelectDriveModeData_Ox420,SelectDriveModeData2_Ox44E,TesterPhysicalResABS_Ox768,TrailerBrakeData_Ox412,WheelData_Ox216,WheelSpeed_Ox217
  wires:
  in_port/1 -> bus_selector/1  "ABS_ESC"
  bus_selector/1 -> ABS_AutoSar_NetworkMgt_Ox596/1(in_port)  "<ABS_AutoSar_NetworkMgt_Ox596>"
  bus_selector/2 -> ABS_BrkBst_Data_Ox4B0/1(in_port)  "<ABS_BrkBst_Data_Ox4B0>"
  bus_selector/3 -> ABS_Rapid_Data_Response_1_Ox6B0/1(in_port)  "<ABS_Rapid_Data_Response_1_Ox6B0>"
  bus_selector/4 -> ABS_Rapid_Data_Response_2_Ox6B1/1(in_port)  "<ABS_Rapid_Data_Response_2_Ox6B1>"
  bus_selector/5 -> ActiveFronSteering_Req_Ox88/1(in_port)  "<ActiveFronSteering_Req_Ox88>"
  bus_selector/6 -> BrakeSnData_3_Ox77/1(in_port)  "<BrakeSnData_3_Ox77>"
  bus_selector/7 -> BrakeSnData_4_Ox7D/1(in_port)  "<BrakeSnData_4_Ox7D>"
  bus_selector/8 -> BrakeSnData_5_Ox76/1(in_port)  "<BrakeSnData_5_Ox76>"
  bus_selector/9 -> BrakeSnData_6_Ox414/1(in_port)  "<BrakeSnData_6_Ox414>"
  bus_selector/10 -> BrakeSysFeatures_Ox415/1(in_port)  "<BrakeSysFeatures_Ox415>"
  bus_selector/11 -> BrakeSysFeatures_2_Ox416/1(in_port)  "<BrakeSysFeatures_2_Ox416>"
  bus_selector/12 -> BrakeSysFeatures_3_Ox41E/1(in_port)  "<BrakeSysFeatures_3_Ox41E>"
  bus_selector/13 -> DesiredTorqBrk_Ox213/1(in_port)  "<DesiredTorqBrk_Ox213>"
  bus_selector/14 -> DesiredTorqBrk_2_Ox214/1(in_port)  "<DesiredTorqBrk_2_Ox214>"
  bus_selector/15 -> Global_PATS_SubTarget_Ox49/1(in_port)  "<Global_PATS_SubTarget_Ox49>"
  bus_selector/16 -> OTAPhysABStoGWM_ECG_Ox1B936028/1(in_port)  "<OTAPhysABStoGWM_ECG_Ox1B936028>"
  bus_selector/17 -> PARSEDPhysABStoGWM_ECG_Ox1BA36028/1(in_port)  "<PARSEDPhysABStoGWM_ECG_Ox1BA36028>"
  bus_selector/18 -> PARSEDPushABStoGWM_ECG_Ox1BB36028/1(in_port)  "<PARSEDPushABStoGWM_ECG_Ox1BB36028>"
  bus_selector/19 -> SelectDriveModeData_Ox420/1(in_port)  "<SelectDriveModeData_Ox420>"
  bus_selector/20 -> SelectDriveModeData2_Ox44E/1(in_port)  "<SelectDriveModeData2_Ox44E>"
  bus_selector/21 -> TesterPhysicalResABS_Ox768/1(in_port)  "<TesterPhysicalResABS_Ox768>"
  bus_selector/22 -> TrailerBrakeData_Ox412/1(in_port)  "<TrailerBrakeData_Ox412>"
  bus_selector/23 -> WheelData_Ox216/1(in_port)  "<WheelData_Ox216>"
  bus_selector/24 -> WheelSpeed_Ox217/1(in_port)  "<WheelSpeed_Ox217>"

== system test_mdl_NI/Subsystem/CMR_DSMC ==
  in_port : Inport
  CMR_DSMC_AutoSar_NetwrkMgt_Ox5DF : Subsystem
  DrvStatMonData_Ox450 : Subsystem
  TesterPhysicalResCMR_DSMC_Ox7C9 : Subsystem
  bus_selector : BusSelector  OutputSignals=CMR_DSMC_AutoSar_NetwrkMgt_Ox5DF,DrvStatMonData_Ox450,TesterPhysicalResCMR_DSMC_Ox7C9
  wires:
  in_port/1 -> bus_selector/1  "CMR_DSMC"
  bus_selector/1 -> CMR_DSMC_AutoSar_NetwrkMgt_Ox5DF/1(in_port)  "<CMR_DSMC_AutoSar_NetwrkMgt_Ox5DF>"
  bus_selector/2 -> DrvStatMonData_Ox450/1(in_port)  "<DrvStatMonData_Ox450>"
  bus_selector/3 -> TesterPhysicalResCMR_DSMC_Ox7C9/1(in_port)  "<TesterPhysicalResCMR_DSMC_Ox7C9>"

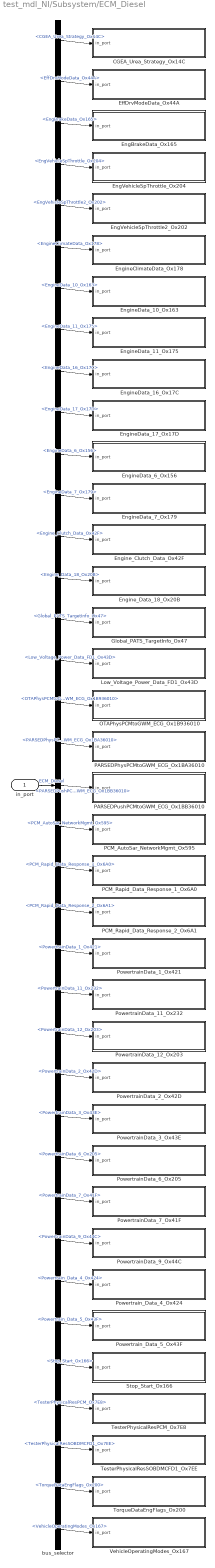
== system test_mdl_NI/Subsystem/ECM_Diesel ==
  in_port : Inport
  CGEA_Urea_Strategy_Ox14C : Subsystem
  EffDrvModeData_Ox44A : Subsystem
  EngBrakeData_Ox165 : Subsystem
  EngVehicleSpThrottle2_Ox202 : Subsystem
  EngVehicleSpThrottle_Ox204 : Subsystem
  EngineClimateData_Ox178 : Subsystem
  EngineData_10_Ox163 : Subsystem
  EngineData_11_Ox175 : Subsystem
  EngineData_16_Ox17C : Subsystem
  EngineData_17_Ox17D : Subsystem
  EngineData_6_Ox156 : Subsystem
  EngineData_7_Ox179 : Subsystem
  Engine_Clutch_Data_Ox42F : Subsystem
  Engine_Data_18_Ox20B : Subsystem
  Global_PATS_TargetInfo_Ox47 : Subsystem
  Low_Voltage_Power_Data_FD1_Ox43D : Subsystem
  OTAPhysPCMtoGWM_ECG_Ox1B936010 : Subsystem
  PARSEDPhysPCMtoGWM_ECG_Ox1BA36010 : Subsystem
  PARSEDPushPCMtoGWM_ECG_Ox1BB36010 : Subsystem
  PCM_AutoSar_NetworkMgmt_Ox595 : Subsystem
  PCM_Rapid_Data_Response_1_Ox6A0 : Subsystem
  PCM_Rapid_Data_Response_2_Ox6A1 : Subsystem
  PowertrainData_11_Ox232 : Subsystem
  PowertrainData_12_Ox203 : Subsystem
  PowertrainData_1_Ox421 : Subsystem
  PowertrainData_2_Ox42D : Subsystem
  PowertrainData_3_Ox43E : Subsystem
  PowertrainData_6_Ox205 : Subsystem
  PowertrainData_7_Ox41F : Subsystem
  PowertrainData_9_Ox44C : Subsystem
  Powertrain_Data_4_Ox424 : Subsystem
  Powertrain_Data_5_Ox43F : Subsystem
  Stop_Start_Ox166 : Subsystem
  TesterPhysicalResPCM_Ox7E8 : Subsystem
  TesterPhysicalResSOBDMCFD1_Ox7EE : Subsystem
  TorqueDataEngFlags_Ox200 : Subsystem
  VehicleOperatingModes_Ox167 : Subsystem
  bus_selector : BusSelector  OutputSignals=CGEA_Urea_Strategy_Ox14C,EffDrvModeData_Ox44A,EngBrakeData_Ox165,EngVehicleSpThrottle_Ox204,EngVehicleSpThrottle2_Ox202,EngineClimateData_Ox178,EngineData_10_Ox163,EngineData_11_Ox175,EngineData_16_Ox17C,EngineData_17_Ox17D,EngineData_6_Ox156,EngineData_7_Ox179,Engine_Clutch_Data_Ox42F,Engine_Data_18_Ox20B,Global_PATS_TargetInfo_Ox47,Low_Voltage_Power_Data_FD1_Ox43D,OTAPhysPCMtoGWM_ECG_Ox1B936010,PARSEDPhysPCMtoGWM_ECG_Ox1BA36010,PARSEDPushPCMtoGWM_ECG_Ox1BB36010,PCM_AutoSar_NetworkMgmt_Ox595,PCM_Rapid_Data_Response_1_Ox6A0,PCM_Rapid_Data_Response_2_Ox6A1,PowertrainData_1_Ox421,PowertrainData_11_Ox232,PowertrainData_12_Ox203,PowertrainData_2_Ox42D,PowertrainData_3_Ox43E,PowertrainData_6_Ox205,PowertrainData_7_Ox41F,PowertrainData_9_Ox44C,Powertrain_Data_4_Ox424,Powertrain_Data_5_Ox43F,Stop_Start_Ox166,TesterPhysicalResPCM_Ox7E8,TesterPhysicalResSOBDMCFD1_Ox7EE,TorqueDataEngFlags_Ox200,VehicleOperatingModes_Ox167
  wires:
  in_port/1 -> bus_selector/1  "ECM_Diesel"
  bus_selector/1 -> CGEA_Urea_Strategy_Ox14C/1(in_port)  "<CGEA_Urea_Strategy_Ox14C>"
  bus_selector/2 -> EffDrvModeData_Ox44A/1(in_port)  "<EffDrvModeData_Ox44A>"
  bus_selector/3 -> EngBrakeData_Ox165/1(in_port)  "<EngBrakeData_Ox165>"
  bus_selector/4 -> EngVehicleSpThrottle_Ox204/1(in_port)  "<EngVehicleSpThrottle_Ox204>"
  bus_selector/5 -> EngVehicleSpThrottle2_Ox202/1(in_port)  "<EngVehicleSpThrottle2_Ox202>"
  bus_selector/6 -> EngineClimateData_Ox178/1(in_port)  "<EngineClimateData_Ox178>"
  bus_selector/7 -> EngineData_10_Ox163/1(in_port)  "<EngineData_10_Ox163>"
  bus_selector/8 -> EngineData_11_Ox175/1(in_port)  "<EngineData_11_Ox175>"
  bus_selector/9 -> EngineData_16_Ox17C/1(in_port)  "<EngineData_16_Ox17C>"
  bus_selector/10 -> EngineData_17_Ox17D/1(in_port)  "<EngineData_17_Ox17D>"
  bus_selector/11 -> EngineData_6_Ox156/1(in_port)  "<EngineData_6_Ox156>"
  bus_selector/12 -> EngineData_7_Ox179/1(in_port)  "<EngineData_7_Ox179>"
  bus_selector/13 -> Engine_Clutch_Data_Ox42F/1(in_port)  "<Engine_Clutch_Data_Ox42F>"
  bus_selector/14 -> Engine_Data_18_Ox20B/1(in_port)  "<Engine_Data_18_Ox20B>"
  bus_selector/15 -> Global_PATS_TargetInfo_Ox47/1(in_port)  "<Global_PATS_TargetInfo_Ox47>"
  bus_selector/16 -> Low_Voltage_Power_Data_FD1_Ox43D/1(in_port)  "<Low_Voltage_Power_Data_FD1_Ox43D>"
  bus_selector/17 -> OTAPhysPCMtoGWM_ECG_Ox1B936010/1(in_port)  "<OTAPhysPCMtoGWM_ECG_Ox1B936010>"
  bus_selector/18 -> PARSEDPhysPCMtoGWM_ECG_Ox1BA36010/1(in_port)  "<PARSEDPhysPCMtoGWM_ECG_Ox1BA36010>"
  bus_selector/19 -> PARSEDPushPCMtoGWM_ECG_Ox1BB36010/1(in_port)  "<PARSEDPushPCMtoGWM_ECG_Ox1BB36010>"
  bus_selector/20 -> PCM_AutoSar_NetworkMgmt_Ox595/1(in_port)  "<PCM_AutoSar_NetworkMgmt_Ox595>"
  bus_selector/21 -> PCM_Rapid_Data_Response_1_Ox6A0/1(in_port)  "<PCM_Rapid_Data_Response_1_Ox6A0>"
  bus_selector/22 -> PCM_Rapid_Data_Response_2_Ox6A1/1(in_port)  "<PCM_Rapid_Data_Response_2_Ox6A1>"
  bus_selector/23 -> PowertrainData_1_Ox421/1(in_port)  "<PowertrainData_1_Ox421>"
  bus_selector/24 -> PowertrainData_11_Ox232/1(in_port)  "<PowertrainData_11_Ox232>"
  bus_selector/25 -> PowertrainData_12_Ox203/1(in_port)  "<PowertrainData_12_Ox203>"
  bus_selector/26 -> PowertrainData_2_Ox42D/1(in_port)  "<PowertrainData_2_Ox42D>"
  bus_selector/27 -> PowertrainData_3_Ox43E/1(in_port)  "<PowertrainData_3_Ox43E>"
  bus_selector/28 -> PowertrainData_6_Ox205/1(in_port)  "<PowertrainData_6_Ox205>"
  bus_selector/29 -> PowertrainData_7_Ox41F/1(in_port)  "<PowertrainData_7_Ox41F>"
  bus_selector/30 -> PowertrainData_9_Ox44C/1(in_port)  "<PowertrainData_9_Ox44C>"
  bus_selector/31 -> Powertrain_Data_4_Ox424/1(in_port)  "<Powertrain_Data_4_Ox424>"
  bus_selector/32 -> Powertrain_Data_5_Ox43F/1(in_port)  "<Powertrain_Data_5_Ox43F>"
  bus_selector/33 -> Stop_Start_Ox166/1(in_port)  "<Stop_Start_Ox166>"
  bus_selector/34 -> TesterPhysicalResPCM_Ox7E8/1(in_port)  "<TesterPhysicalResPCM_Ox7E8>"
  bus_selector/35 -> TesterPhysicalResSOBDMCFD1_Ox7EE/1(in_port)  "<TesterPhysicalResSOBDMCFD1_Ox7EE>"
  bus_selector/36 -> TorqueDataEngFlags_Ox200/1(in_port)  "<TorqueDataEngFlags_Ox200>"
  bus_selector/37 -> VehicleOperatingModes_Ox167/1(in_port)  "<VehicleOperatingModes_Ox167>"
